simulink model "sampleModel211"  (R2021b)
settings: Solver=VariableStepAuto  StartTime=0.0  StopTime=10.0  RelTol=1e-3
undefined symbols (not defined in the file or in its folder): Newton, Raphson
libraries: simulink x7
settings Model: Creator=user  LastModifiedBy=user

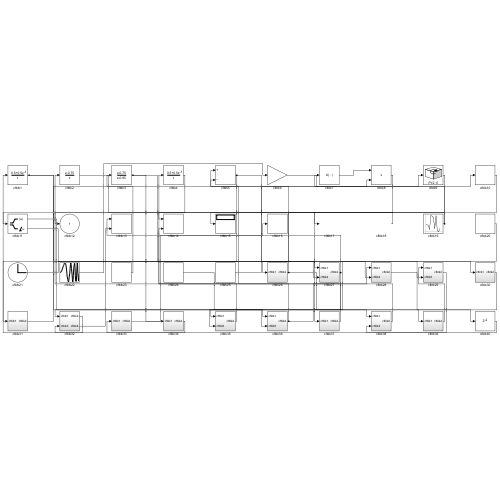
[thumbnail: Simulink's stored preview of the top-level diagram]
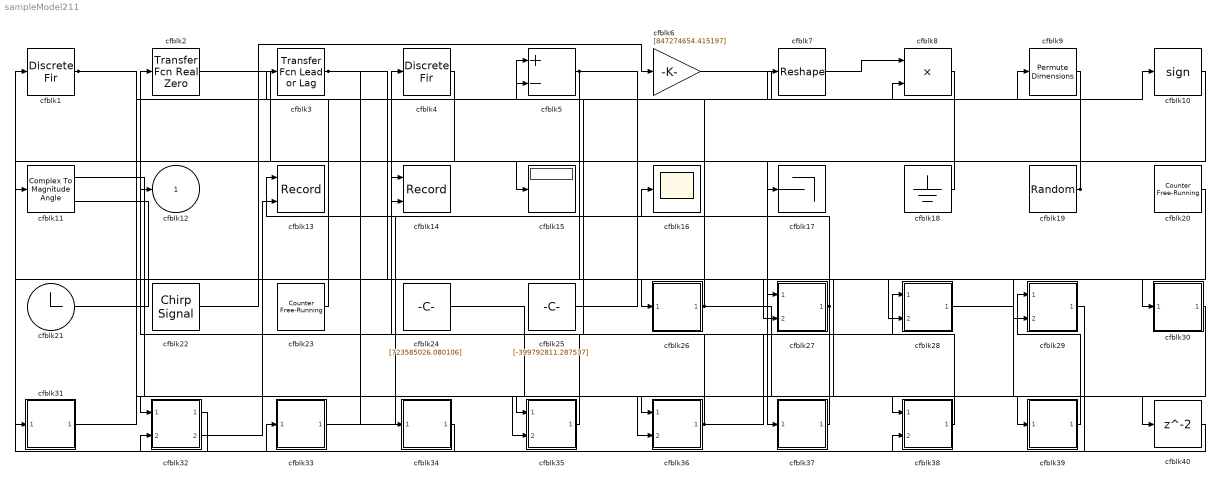
== system sampleModel211 ==
  cfblk1 : DiscreteFir  SampleTime=1
  cfblk10 : Signum
  cfblk11 : ComplexToMagnitudeAngle
  cfblk13 : Record  FileSettingsInternal="{\"entries\":[{\"content\":{\"excelSettings\":{\"content\":{},\"type\":\"Streamout.ExcelSettings\"}},\"type\":\"Streamout.FileSettingStorage\",\"uuid\":\"afcd1033-900c-4ee9-9df4-e3060ae59736\"}],\"packageUris\":[\"http://schema.mathworks.com/mf0/streamout_blocks/R2020a\"],\"version\":\"1.0\"}"  Layout=[1 1]  SignalsInternal="{\"entries\":[{\"content\":{\"signals\":[{\"content\":{\"blockPath\":[\"sampleModel211/cfblk13\"],\"channel\":[],\"dimensions\":[1],\"domain\":\"sampleModel211/cfblk13\",\"lineColor\":\"#a2142f\",\"plots\":[1],\"port\":1,\"sid\":[\"\"],\"signalID\":8172,\"signalName\":\"cfblk27\"},\"type\":\"RecordBlkView.Signal\",\"uuid\":\"39aa8972-9eb6-4579-9132-f180a06a49c1\"},{\"content\":{\"blockPath\":[\"sampleModel211/cfblk13\"],\"channel\":[],\"dimensions\":[1],\"domain\":\"sampleModel211/cfblk13\",\"lineColor\":\"#139fff\",\"plots\":[1],\"port\":2,\"sid\":[\"\"],\"signalID\":8178,\"signalName\":\"cfblk32:2\"},\"type\":\"RecordBlkView.Signal\",\"uuid\":\"5eb831b9-ae7c-4887-863b-56d573ecb515\"}]},\"type\":\"RecordBlkView.InputSignals\",\"uuid\":\"4502b0b9-b198-4663-ab9e-d3e6dd85faee\"}],\"packageUris\":[\"http://schema.mathworks.com/mf0/streamout_blocks/R2020a\"],\"version\":\"1.0\"}"  VisualizationBindings="{\"xyplotplugin\":{\"info\":[{\"series\":[{\"bindingParametersList\":[{\"parameter\":\"X-Axis\",\"signalID\":8172,\"signalName\":\"cfblk27\"},{\"parameter\":\"Y-Axis\",\"signalID\":8178,\"signalName\":\"cfblk32:2\"}],\"seriesID\":42711}],\"subplotID\":1}]}}"  CompatibilityTag=XY
  cfblk14 : Record  FileSettingsInternal="{\"entries\":[{\"content\":{\"excelSettings\":{\"content\":{},\"type\":\"Streamout.ExcelSettings\"}},\"type\":\"Streamout.FileSettingStorage\",\"uuid\":\"20000c39-0e0b-4ded-a58f-0152ac3ac14a\"}],\"packageUris\":[\"http://schema.mathworks.com/mf0/streamout_blocks/R2020a\"],\"version\":\"1.0\"}"  Layout=[1 1]  SignalsInternal="{\"entries\":[{\"content\":{\"signals\":[{\"content\":{\"blockPath\":[\"sampleModel211/cfblk14\"],\"channel\":[],\"dimensions\":[1],\"domain\":\"sampleModel211/cfblk14\",\"lineColor\":\"#139fff\",\"plots\":[1],\"port\":2,\"sid\":[\"\"],\"signalID\":8182,\"signalName\":\"cfblk36\"},\"type\":\"RecordBlkView.Signal\",\"uuid\":\"7c038ca0-a94d-4e51-8edb-2469e55715a0\"},{\"content\":{\"blockPath\":[\"sampleModel211/cfblk14\"],\"channel\":[],\"dimensions\":[1],\"domain\":\"sampleModel211/cfblk14\",\"lineColor\":\"#a2142f\",\"plots\":[1],\"port\":1,\"sid\":[\"\"],\"signalID\":8186,\"signalName\":\"cfblk18\"},\"type\":\"RecordBlkView.Signal\",\"uuid\":\"c3ed6209-edfc-4510-8781-c1ae4b83dc9e\"}]},\"type\":\"RecordBlkView.InputSignals\",\"uuid\":\"187a8363-9b1c-4df1-b857-5c764666650c\"}],\"packageUris\":[\"http://schema.mathworks.com/mf0/streamout_blocks/R2020a\"],\"version\":\"1.0\"}"  VisualizationBindings="{\"xyplotplugin\":{\"info\":[{\"series\":[{\"bindingParametersList\":[{\"parameter\":\"X-Axis\",\"signalID\":8186,\"signalName\":\"cfblk18\"},{\"parameter\":\"Y-Axis\",\"signalID\":8182,\"signalName\":\"cfblk36\"}],\"seriesID\":19308}],\"subplotID\":1}]}}"  CompatibilityTag=XY
  cfblk15 : Display
  cfblk16 : Scope
  cfblk17 : Terminator
  cfblk18 : Ground
  cfblk19 : RandomNumber  Mean=[89903.066414]  Variance=[37427.790847]  Seed=[18408499.000000]  SampleTime=0.1
  cfblk2 : simulink/Discrete/Transfer Fcn Real Zero  ZeroZ=0.75  ICPrevInput=0.0  DoSatur=off
      settings: SourceProductBaseCode=SL
  cfblk20 : simulink/Sources/Counter Free-Running  NumBits=[15.000000]  tsamp=-1
  cfblk21 : Clock
  cfblk22 : simulink/Sources/Chirp Signal  f1=[-913289439.789139]  T=[-730390631.039313]  f2=[32941543.814136]
  cfblk23 : simulink/Sources/Counter Free-Running  NumBits=[12.000000]  tsamp=-1
  cfblk24 : Constant  Value=[723585026.080106]  SampleTime=1
  cfblk25 : Constant  Value=[-399792811.287537]  SampleTime=1
  cfblk26 : Subsystem
  cfblk27 : Subsystem
  cfblk28 : Subsystem
  cfblk29 : Subsystem
  cfblk3 : simulink/Discrete/Transfer Fcn Lead or Lag  PoleZ=0.95  ZeroZ=0.75  ICPrevOutput=0.0  ICPrevInput=0.0  DoSatur=off
      settings: SourceProductBaseCode=SL
  cfblk30 : Subsystem
  cfblk31 : Subsystem
  cfblk32 : Subsystem
  cfblk33 : Subsystem
  cfblk34 : Subsystem
  cfblk35 : Subsystem
  cfblk36 : Subsystem
  cfblk37 : Subsystem
  cfblk38 : Subsystem
  cfblk39 : Subsystem
  cfblk4 : DiscreteFir  SampleTime=1
  cfblk40 : Delay  SampleTime=1
  cfblk5 : Sum  Inputs=+-
  cfblk6 : Gain  Gain=[847274654.415197]
  cfblk7 : Reshape
  cfblk8 : Product  Inputs=**
  cfblk9 : PermuteDimensions
  cfblk12 : Outport
  wires:
  cfblk27/1(cfblk2) -> cfblk13/1, cfblk35/2(cfblk5)
  cfblk20/1 -> cfblk32/1(cfblk1)
  cfblk37/1(cfblk2) -> cfblk4/1
  cfblk33/1(cfblk2) -> cfblk16/1
  cfblk32/1(cfblk2) -> cfblk1/1
  cfblk22/1 -> cfblk6/1
  cfblk26/1(cfblk2) -> cfblk39/1(cfblk1), cfblk5/2
  cfblk29/1(cfblk2) -> cfblk33/1(cfblk1)
  cfblk7/1 -> cfblk8/1
  cfblk35/1(cfblk2) -> cfblk2/1
  cfblk5/1 -> cfblk31/1(cfblk1), cfblk28/2(cfblk4)
  cfblk32/2(cfblk4) -> cfblk13/2
  cfblk10/1 -> cfblk37/1(cfblk1)
  cfblk30/1(cfblk2) -> cfblk35/1(cfblk1)
  cfblk4/1 -> cfblk11/1
  cfblk9/1 -> cfblk26/1(cfblk1)
  cfblk34/1(cfblk2) -> cfblk32/2(cfblk3)
  cfblk39/1(cfblk2) -> cfblk29/1(cfblk1)
  cfblk31/1(cfblk2) -> cfblk10/1
  cfblk25/1 -> cfblk9/1
  cfblk3/1 -> cfblk29/2(cfblk5), cfblk34/1(cfblk1)
  cfblk36/1(cfblk2) -> cfblk28/1(cfblk1), cfblk14/2
  cfblk11/1 -> cfblk36/1(cfblk1)
  cfblk18/1 -> cfblk14/1
  cfblk21/1 -> cfblk30/1(cfblk1)
  cfblk1/1 -> cfblk38/1(cfblk1), cfblk27/2(cfblk4)
  cfblk6/1 -> cfblk8/2
  cfblk24/1 -> cfblk36/2(cfblk5)
  cfblk11/2 -> cfblk27/1(cfblk1)
  cfblk8/1 -> cfblk15/1
  cfblk19/1 -> cfblk7/1, cfblk12/1
  cfblk38/1(cfblk2) -> cfblk5/1
  cfblk2/1 -> cfblk17/1
  cfblk23/1 -> cfblk3/1
  cfblk28/1(cfblk2) -> cfblk40/1
  cfblk40/1 -> cfblk38/2(cfblk4)

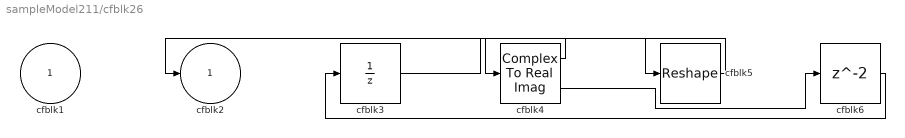
== system sampleModel211/cfblk26 ==
  cfblk1 : Inport
  cfblk3 : UnitDelay  HasFrameUpgradeWarning=on
  cfblk4 : ComplexToRealImag
  cfblk5 : Reshape
  cfblk6 : Delay  SampleTime=1
  cfblk2 : Outport
  wires:
  cfblk4/1 -> cfblk2/1
  cfblk5/1 -> cfblk4/1
  cfblk3/1 -> cfblk5/1
  cfblk4/2 -> cfblk6/1
  cfblk6/1 -> cfblk3/1

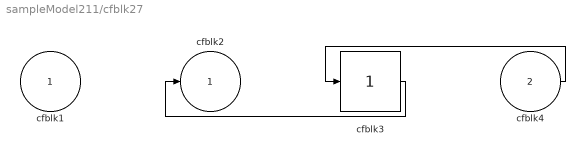
== system sampleModel211/cfblk27 ==
  cfblk1 : Inport
  cfblk4 : Inport  Port=2
  cfblk3 : simulink/Math Operations/Slider Gain  gain=1  low=0  high=2
  cfblk2 : Outport
  wires:
  cfblk4/1 -> cfblk3/1
  cfblk3/1 -> cfblk2/1

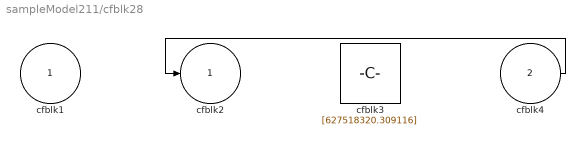
== system sampleModel211/cfblk28 ==
  cfblk1 : Inport
  cfblk4 : Inport  Port=2
  cfblk3 : Constant  Value=[627518320.309116]  SampleTime=1
  cfblk2 : Outport
  wires:
  cfblk4/1 -> cfblk2/1

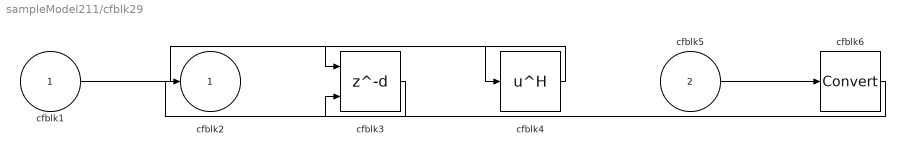
== system sampleModel211/cfblk29 ==
  cfblk1 : Inport
  cfblk5 : Inport  Port=2
  cfblk3 : Delay  DelayLengthSource=Input port  SampleTime=1
      settings: InputPortMap=u0,p1
  cfblk4 : Math  Operator=hermitian  SaturateOnIntegerOverflow=on
  cfblk6 : DataTypeConversion
  cfblk2 : Outport
  wires:
  cfblk1/1 -> cfblk4/1
  cfblk3/1 -> cfblk2/1
  cfblk4/1 -> cfblk3/1
  cfblk5/1 -> cfblk6/1
  cfblk6/1 -> cfblk3/2

== system sampleModel211/cfblk30 ==
  cfblk1 : Inport
  cfblk3 : UnaryMinus
  cfblk2 : Outport
  wires:
  cfblk1/1 -> cfblk3/1
  cfblk3/1 -> cfblk2/1

== system sampleModel211/cfblk31 ==
  cfblk1 : Inport
  cfblk3 : UnitDelay  HasFrameUpgradeWarning=on
  cfblk2 : Outport
  wires:
  cfblk3/1 -> cfblk2/1
  cfblk1/1 -> cfblk3/1

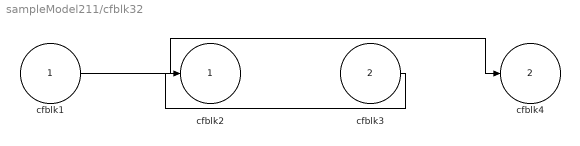
== system sampleModel211/cfblk32 ==
  cfblk1 : Inport
  cfblk3 : Inport  Port=2
  cfblk2 : Outport
  cfblk4 : Outport  Port=2
  wires:
  cfblk1/1 -> cfblk4/1
  cfblk3/1 -> cfblk2/1

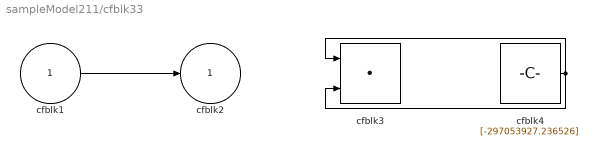
== system sampleModel211/cfblk33 ==
  cfblk1 : Inport
  cfblk3 : DotProduct  InputSameDT=on  OutDataTypeStr=Inherit: Inherit via internal rule
  cfblk4 : Constant  Value=[-297053927.236526]  SampleTime=1
  cfblk2 : Outport
  wires:
  cfblk4/1 -> cfblk3/1, cfblk3/2
  cfblk1/1 -> cfblk2/1

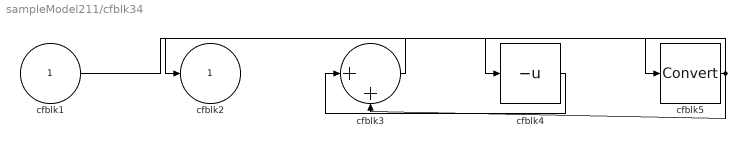
== system sampleModel211/cfblk34 ==
  cfblk1 : Inport
  cfblk3 : Sum  Inputs=|++
  cfblk4 : UnaryMinus
  cfblk5 : DataTypeConversion
  cfblk2 : Outport
  wires:
  cfblk3/1 -> cfblk2/1
  cfblk4/1 -> cfblk3/1
  cfblk1/1 -> cfblk5/1
  cfblk5/1 -> cfblk4/1, cfblk3/2

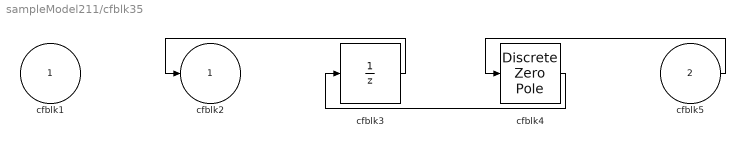
== system sampleModel211/cfblk35 ==
  cfblk1 : Inport
  cfblk5 : Inport  Port=2
  cfblk3 : UnitDelay  HasFrameUpgradeWarning=on
  cfblk4 : DiscreteZeroPole  Poles=[0 0.5]  Gain=1
  cfblk2 : Outport
  wires:
  cfblk5/1 -> cfblk4/1
  cfblk3/1 -> cfblk2/1
  cfblk4/1 -> cfblk3/1

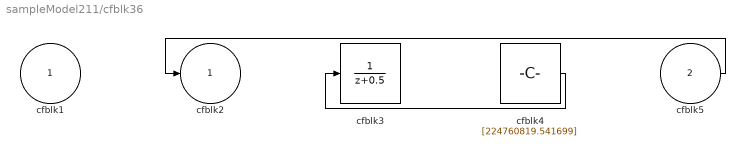
== system sampleModel211/cfblk36 ==
  cfblk1 : Inport
  cfblk5 : Inport  Port=2
  cfblk3 : DiscreteTransferFcn  SampleTime=1
  cfblk4 : Constant  Value=[224760819.541699]  SampleTime=1
  cfblk2 : Outport
  wires:
  cfblk5/1 -> cfblk2/1
  cfblk4/1 -> cfblk3/1

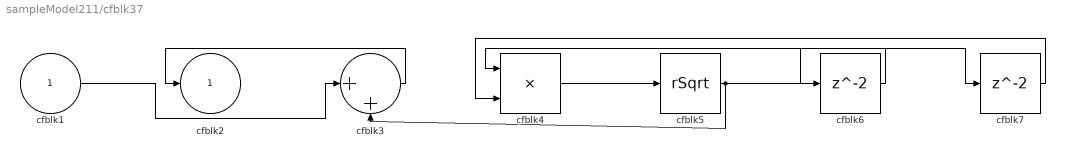
== system sampleModel211/cfblk37 ==
  cfblk1 : Inport
  cfblk3 : Sum  Inputs=|++
  cfblk4 : Product  Inputs=**
  cfblk5 : Sqrt  Operator=rSqrt  AlgorithmType=Newton-Raphson  SaturateOnIntegerOverflow=on
  cfblk6 : Delay  SampleTime=1
  cfblk7 : Delay  SampleTime=1
  cfblk2 : Outport
  wires:
  cfblk3/1 -> cfblk2/1
  cfblk4/1 -> cfblk5/1
  cfblk1/1 -> cfblk3/1
  cfblk5/1 -> cfblk3/2, cfblk6/1, cfblk7/1
  cfblk6/1 -> cfblk4/1
  cfblk7/1 -> cfblk4/2

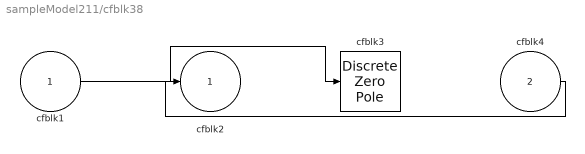
== system sampleModel211/cfblk38 ==
  cfblk1 : Inport
  cfblk4 : Inport  Port=2
  cfblk3 : DiscreteZeroPole  Poles=[0 0.5]  Gain=1
  cfblk2 : Outport
  wires:
  cfblk1/1 -> cfblk3/1
  cfblk4/1 -> cfblk2/1

== system sampleModel211/cfblk39 ==
  cfblk1 : Inport
  cfblk3 : simulink/Discrete/Difference  ICPrevInput=0.0  OutMin=[]  OutMax=[]  OutDataTypeStr=Inherit: Inherit via back propagation  OutDataType=fixdt(1, 16)  OutScaling=2^-10  DoSatur=off
  cfblk2 : Outport
  wires:
  cfblk1/1 -> cfblk3/1
  cfblk3/1 -> cfblk2/1
